simulink model "chap02_63"  (R2013b)
settings: Solver=ode45  StartTime=0.0  StopTime=10.0  RelTol=1e-3
libraries: dspsrcs4 x1
settings Model: Creator=Administrator  LastModifiedBy=sunzx.fnst

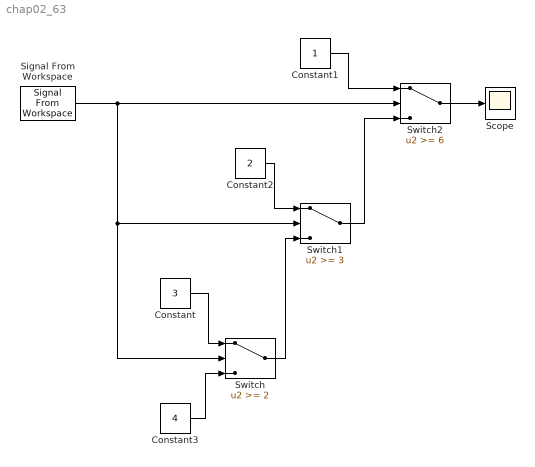
== system chap02_63 ==
  Constant : Constant  Value=3
  Constant1 : Constant
  Constant2 : Constant  Value=2
  Constant3 : Constant  Value=4
  Scope : Scope
  Signal From Workspace : dspsrcs4/Signal From Workspace  X=0:10  Ts=1  nsamps=1  OutputAfterFinalValue=Setting to zero  ignoreOrWarnInputAndFrameLengths=off
  Switch : Switch  Threshold=2
      settings: AttributesFormatString=Threshold = %<Threshold>
  Switch1 : Switch  Threshold=3
      settings: AttributesFormatString=Threshold = %<Threshold>
  Switch2 : Switch  Threshold=6
      settings: AttributesFormatString=Threshold = %<Threshold>
  wires:
  Signal From Workspace/1 -> Switch/2, Switch1/2, Switch2/2
  Constant1/1 -> Switch2/1
  Switch1/1 -> Switch2/3
  Switch2/1 -> Scope/1
  Constant2/1 -> Switch1/1
  Switch/1 -> Switch1/3
  Constant/1 -> Switch/1
  Constant3/1 -> Switch/3
